simulink model "BatteryFarmTemplate"  (R2022b)
settings: Solver=VariableStepAuto  StartTime=0.0  StopTime=10.0  RelTol=1e-3  AbsTol=1e-3  EnableMultiTasking=on
libraries: ee_lib x242, sdl_lib x84, fl_lib x43
(part 1 of 5)
settings Model: Creator=Kimberly1!  LastModifiedBy=minar
settings SolverCC: AutoScaleAbsTol=off  AlgebraicLoopSolver=TrustRegion  MaxZcPerStep=1
settings DataIOCC: LimitDataPoints=on  MaxDataPoints=10000
settings OptimizationCC: LifeSpan=inf
settings DebuggingCC: UnconnectedInputMsg=warning  UnconnectedOutputMsg=warning  UnconnectedLineMsg=warning  AllowSymbolicDim=off  SFUnexpectedBacktrackingDiag=warning  SFNoUnconditionalDefaultTransitionDiag=warning  SFExecutionAtInitializationDiag=none  SFMachineParentedDataDiag=warning  ArithmeticOperatorsInVariantConditions=warning
settings ModelReferenceCC: EnableRefExpFcnMdlSchedulingChecks=on
settings SFSimCC: SimUseLocalCustomCode=off  CustomCodeUndefinedFunction=UseInterfaceOnly
settings RTWCC: RTWUseLocalCustomCode=off  DLArmComputeVersion=19.05
settings CodeAppCC: StateflowObjectComments=on
settings GRTTargetCC: TargetLangStandard=C89/C90 (ANSI)
settings ConfigComp: CovMetricSettings=dw  CovSaveCumulativeToWorkspaceVar=on  CovSaveSingleToWorkspaceVar=on  CovExternalEMLEnable=off  CovSFcnEnable=off
settings SimscapeCC: SimscapeLogType=all  SimscapeLogSimulationStatistics=on  SimscapeLogDataHistory=10000

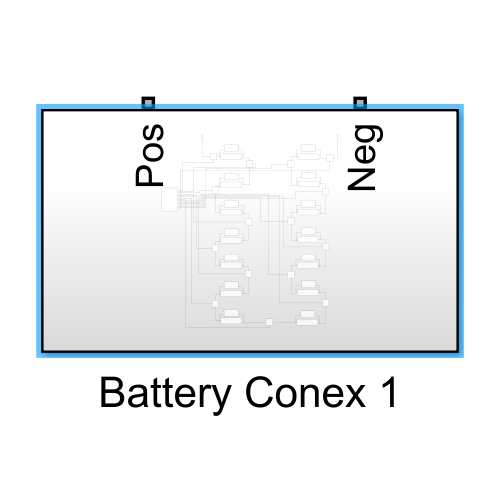
[thumbnail: Simulink's stored preview of the top-level diagram]
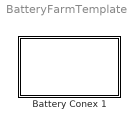
== system BatteryFarmTemplate ==
  Battery Conex 1 : Subsystem
      settings: PortSchema="{\"entries\":[{\"content\":{\"sides\":[{\"content\":{\"connectorIds\":[]},\"type\":\"ConnectorPlacement.EquallySpacedRectSide\",\"uuid\":\"048fa1c2-ad06-4d9f-ba7c-aee5a0b8c9f2\"},{\"content\":{\"connectorIds\":[],\"side\":\"RIGHT\"},\"type\":\"ConnectorPlacement.EquallySpacedRectSide\",\"uuid\":\"f15e2629-eceb-4a27-921b-d8c57562cf10\"},{\"content\":{\"connectorIds\":[\"LConn1\",\"LConn2\"],\"side\":\"TOP\"},\"type\":\"ConnectorPlacement.EquallySpacedRectSide\",\"uuid\":\"4da660f4-bcfa-4f4c-af01-21485ad5be59\"}]},\"type\":\"ConnectorPlacement.EquallySpacedConnector\",\"uuid\":\"40cf05ef-0db3-4ef6-b98b-cb586730e4e3\"}],\"packageUris\":[\"http://schema.mathworks.com/mf0/Connector/R2020b\"],\"version\":\"1.0\"}"

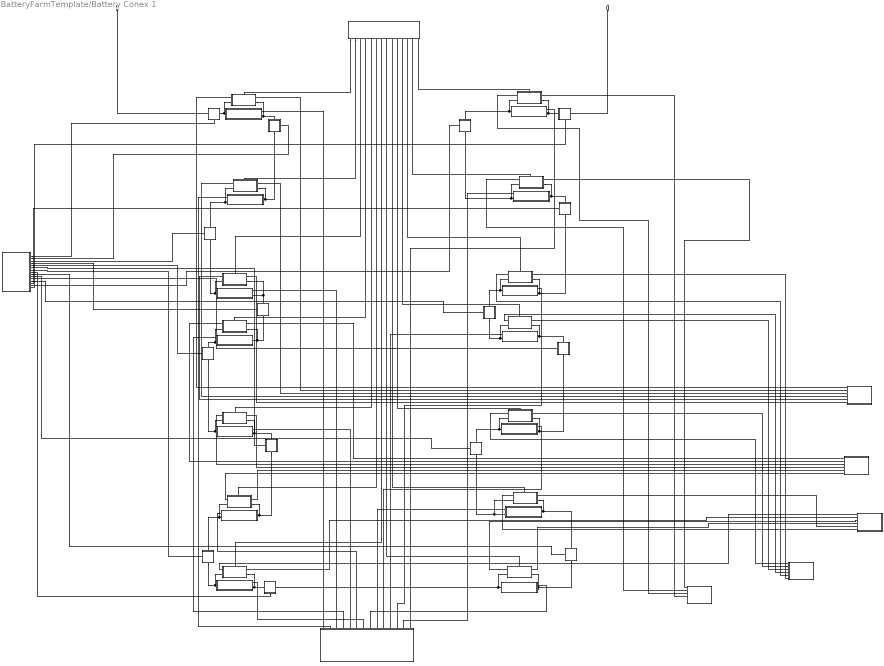
== system BatteryFarmTemplate/Battery Conex 1 ==
  Battery Charger 1 : Subsystem
  Battery Charger 2 : Subsystem
  Battery Charger 3 : Subsystem
  Battery Charger 4 : Subsystem
  Battery Charger 5 : Subsystem
  Battery Module 1 : Subsystem
  Battery Module 10 : Subsystem
  Battery Module 11 : Subsystem
  Battery Module 12 : Subsystem
  Battery Module 13 : Subsystem
  Battery Module 14 : Subsystem
  Battery Module 2 : Subsystem
  Battery Module 3 : Subsystem
  Battery Module 4 : Subsystem
  Battery Module 5 : Subsystem
  Battery Module 6 : Subsystem
  Battery Module 7 : Subsystem
  Battery Module 8 : Subsystem
  Battery Module 9 : Subsystem
  Busbar  SW 1 : Subsystem
      settings: PortSchema="{\"entries\":[{\"content\":{\"sides\":[{\"content\":{\"connectorIds\":[\"LConn1\"]},\"type\":\"ConnectorPlacement.EquallySpacedRectSide\",\"uuid\":\"9cfb2e44-9dde-4df9-b010-27803d6f9c91\"},{\"content\":{\"connectorIds\":[\"RConn1\"],\"side\":\"RIGHT\"},\"type\":\"ConnectorPlacement.EquallySpacedRectSide\",\"uuid\":\"4d379f47-42d8-42e3-9ed0-68a717690785\"},{\"content\":{\"connectorIds\":[],\"side\":\"TOP\"},\"type\":\"ConnectorPlacement.EquallySpacedRectSide\",\"uuid\":\"04b3dae9-36fd-4179-bf2b-fdf6296dfe4e\"},{\"content\":{\"connectorIds\":[\"RConn2\"],\"side\":\"BOTTOM\"},\"type\":\"ConnectorPlacement.EquallySpacedRectSide\",\"uuid\":\"a7774700-76cb-4b6b-87b6-7d3fc687af73\"}]},\"type\":\"ConnectorPlacement.EquallySpacedConnector\",\"uuid\":\"06353b4d-18ff-4963-8ee5-abf5474e4c27\"}],\"packageUris\":[\"http://schema.mathworks.com/mf0/Connector/R2020b\"],\"version\":\"1.0\"}"
  Busbar  SW 10 : Subsystem
      settings: PortSchema="{\"entries\":[{\"content\":{\"sides\":[{\"content\":{\"connectorIds\":[\"LConn1\"]},\"type\":\"ConnectorPlacement.EquallySpacedRectSide\",\"uuid\":\"9cfb2e44-9dde-4df9-b010-27803d6f9c91\"},{\"content\":{\"connectorIds\":[\"RConn1\"],\"side\":\"RIGHT\"},\"type\":\"ConnectorPlacement.EquallySpacedRectSide\",\"uuid\":\"4d379f47-42d8-42e3-9ed0-68a717690785\"},{\"content\":{\"connectorIds\":[],\"side\":\"TOP\"},\"type\":\"ConnectorPlacement.EquallySpacedRectSide\",\"uuid\":\"04b3dae9-36fd-4179-bf2b-fdf6296dfe4e\"},{\"content\":{\"connectorIds\":[\"RConn2\"],\"side\":\"BOTTOM\"},\"type\":\"ConnectorPlacement.EquallySpacedRectSide\",\"uuid\":\"a7774700-76cb-4b6b-87b6-7d3fc687af73\"}]},\"type\":\"ConnectorPlacement.EquallySpacedConnector\",\"uuid\":\"06353b4d-18ff-4963-8ee5-abf5474e4c27\"}],\"packageUris\":[\"http://schema.mathworks.com/mf0/Connector/R2020b\"],\"version\":\"1.0\"}"
  Busbar  SW 11 : Subsystem
      settings: PortSchema="{\"entries\":[{\"content\":{\"sides\":[{\"content\":{\"connectorIds\":[\"LConn1\"]},\"type\":\"ConnectorPlacement.EquallySpacedRectSide\",\"uuid\":\"9cfb2e44-9dde-4df9-b010-27803d6f9c91\"},{\"content\":{\"connectorIds\":[\"RConn1\"],\"side\":\"RIGHT\"},\"type\":\"ConnectorPlacement.EquallySpacedRectSide\",\"uuid\":\"4d379f47-42d8-42e3-9ed0-68a717690785\"},{\"content\":{\"connectorIds\":[],\"side\":\"TOP\"},\"type\":\"ConnectorPlacement.EquallySpacedRectSide\",\"uuid\":\"04b3dae9-36fd-4179-bf2b-fdf6296dfe4e\"},{\"content\":{\"connectorIds\":[\"RConn2\"],\"side\":\"BOTTOM\"},\"type\":\"ConnectorPlacement.EquallySpacedRectSide\",\"uuid\":\"a7774700-76cb-4b6b-87b6-7d3fc687af73\"}]},\"type\":\"ConnectorPlacement.EquallySpacedConnector\",\"uuid\":\"06353b4d-18ff-4963-8ee5-abf5474e4c27\"}],\"packageUris\":[\"http://schema.mathworks.com/mf0/Connector/R2020b\"],\"version\":\"1.0\"}"
  Busbar  SW 12 : Subsystem
      settings: PortSchema="{\"entries\":[{\"content\":{\"sides\":[{\"content\":{\"connectorIds\":[\"LConn1\"]},\"type\":\"ConnectorPlacement.EquallySpacedRectSide\",\"uuid\":\"9cfb2e44-9dde-4df9-b010-27803d6f9c91\"},{\"content\":{\"connectorIds\":[\"RConn1\"],\"side\":\"RIGHT\"},\"type\":\"ConnectorPlacement.EquallySpacedRectSide\",\"uuid\":\"4d379f47-42d8-42e3-9ed0-68a717690785\"},{\"content\":{\"connectorIds\":[],\"side\":\"TOP\"},\"type\":\"ConnectorPlacement.EquallySpacedRectSide\",\"uuid\":\"04b3dae9-36fd-4179-bf2b-fdf6296dfe4e\"},{\"content\":{\"connectorIds\":[\"RConn2\"],\"side\":\"BOTTOM\"},\"type\":\"ConnectorPlacement.EquallySpacedRectSide\",\"uuid\":\"a7774700-76cb-4b6b-87b6-7d3fc687af73\"}]},\"type\":\"ConnectorPlacement.EquallySpacedConnector\",\"uuid\":\"06353b4d-18ff-4963-8ee5-abf5474e4c27\"}],\"packageUris\":[\"http://schema.mathworks.com/mf0/Connector/R2020b\"],\"version\":\"1.0\"}"
  Busbar  SW 13 : Subsystem
      settings: PortSchema="{\"entries\":[{\"content\":{\"sides\":[{\"content\":{\"connectorIds\":[\"LConn1\"]},\"type\":\"ConnectorPlacement.EquallySpacedRectSide\",\"uuid\":\"9cfb2e44-9dde-4df9-b010-27803d6f9c91\"},{\"content\":{\"connectorIds\":[\"RConn1\"],\"side\":\"RIGHT\"},\"type\":\"ConnectorPlacement.EquallySpacedRectSide\",\"uuid\":\"4d379f47-42d8-42e3-9ed0-68a717690785\"},{\"content\":{\"connectorIds\":[],\"side\":\"TOP\"},\"type\":\"ConnectorPlacement.EquallySpacedRectSide\",\"uuid\":\"04b3dae9-36fd-4179-bf2b-fdf6296dfe4e\"},{\"content\":{\"connectorIds\":[\"RConn2\"],\"side\":\"BOTTOM\"},\"type\":\"ConnectorPlacement.EquallySpacedRectSide\",\"uuid\":\"a7774700-76cb-4b6b-87b6-7d3fc687af73\"}]},\"type\":\"ConnectorPlacement.EquallySpacedConnector\",\"uuid\":\"06353b4d-18ff-4963-8ee5-abf5474e4c27\"}],\"packageUris\":[\"http://schema.mathworks.com/mf0/Connector/R2020b\"],\"version\":\"1.0\"}"
  Busbar  SW 14 : Subsystem
      settings: PortSchema="{\"entries\":[{\"content\":{\"sides\":[{\"content\":{\"connectorIds\":[\"LConn1\"]},\"type\":\"ConnectorPlacement.EquallySpacedRectSide\",\"uuid\":\"9cfb2e44-9dde-4df9-b010-27803d6f9c91\"},{\"content\":{\"connectorIds\":[\"RConn1\"],\"side\":\"RIGHT\"},\"type\":\"ConnectorPlacement.EquallySpacedRectSide\",\"uuid\":\"4d379f47-42d8-42e3-9ed0-68a717690785\"},{\"content\":{\"connectorIds\":[],\"side\":\"TOP\"},\"type\":\"ConnectorPlacement.EquallySpacedRectSide\",\"uuid\":\"04b3dae9-36fd-4179-bf2b-fdf6296dfe4e\"},{\"content\":{\"connectorIds\":[\"RConn2\"],\"side\":\"BOTTOM\"},\"type\":\"ConnectorPlacement.EquallySpacedRectSide\",\"uuid\":\"a7774700-76cb-4b6b-87b6-7d3fc687af73\"}]},\"type\":\"ConnectorPlacement.EquallySpacedConnector\",\"uuid\":\"06353b4d-18ff-4963-8ee5-abf5474e4c27\"}],\"packageUris\":[\"http://schema.mathworks.com/mf0/Connector/R2020b\"],\"version\":\"1.0\"}"
  Busbar  SW 15 : Subsystem
      settings: PortSchema="{\"entries\":[{\"content\":{\"sides\":[{\"content\":{\"connectorIds\":[\"LConn1\"]},\"type\":\"ConnectorPlacement.EquallySpacedRectSide\",\"uuid\":\"9cfb2e44-9dde-4df9-b010-27803d6f9c91\"},{\"content\":{\"connectorIds\":[\"RConn1\"],\"side\":\"RIGHT\"},\"type\":\"ConnectorPlacement.EquallySpacedRectSide\",\"uuid\":\"4d379f47-42d8-42e3-9ed0-68a717690785\"},{\"content\":{\"connectorIds\":[],\"side\":\"TOP\"},\"type\":\"ConnectorPlacement.EquallySpacedRectSide\",\"uuid\":\"04b3dae9-36fd-4179-bf2b-fdf6296dfe4e\"},{\"content\":{\"connectorIds\":[\"RConn2\"],\"side\":\"BOTTOM\"},\"type\":\"ConnectorPlacement.EquallySpacedRectSide\",\"uuid\":\"a7774700-76cb-4b6b-87b6-7d3fc687af73\"}]},\"type\":\"ConnectorPlacement.EquallySpacedConnector\",\"uuid\":\"06353b4d-18ff-4963-8ee5-abf5474e4c27\"}],\"packageUris\":[\"http://schema.mathworks.com/mf0/Connector/R2020b\"],\"version\":\"1.0\"}"
  Busbar  SW 2 : Subsystem
      settings: PortSchema="{\"entries\":[{\"content\":{\"sides\":[{\"content\":{\"connectorIds\":[\"LConn1\"]},\"type\":\"ConnectorPlacement.EquallySpacedRectSide\",\"uuid\":\"9cfb2e44-9dde-4df9-b010-27803d6f9c91\"},{\"content\":{\"connectorIds\":[\"RConn1\"],\"side\":\"RIGHT\"},\"type\":\"ConnectorPlacement.EquallySpacedRectSide\",\"uuid\":\"4d379f47-42d8-42e3-9ed0-68a717690785\"},{\"content\":{\"connectorIds\":[],\"side\":\"TOP\"},\"type\":\"ConnectorPlacement.EquallySpacedRectSide\",\"uuid\":\"04b3dae9-36fd-4179-bf2b-fdf6296dfe4e\"},{\"content\":{\"connectorIds\":[\"RConn2\"],\"side\":\"BOTTOM\"},\"type\":\"ConnectorPlacement.EquallySpacedRectSide\",\"uuid\":\"a7774700-76cb-4b6b-87b6-7d3fc687af73\"}]},\"type\":\"ConnectorPlacement.EquallySpacedConnector\",\"uuid\":\"06353b4d-18ff-4963-8ee5-abf5474e4c27\"}],\"packageUris\":[\"http://schema.mathworks.com/mf0/Connector/R2020b\"],\"version\":\"1.0\"}"
  Busbar  SW 3 : Subsystem
      settings: PortSchema="{\"entries\":[{\"content\":{\"sides\":[{\"content\":{\"connectorIds\":[\"LConn1\"]},\"type\":\"ConnectorPlacement.EquallySpacedRectSide\",\"uuid\":\"9cfb2e44-9dde-4df9-b010-27803d6f9c91\"},{\"content\":{\"connectorIds\":[\"RConn1\"],\"side\":\"RIGHT\"},\"type\":\"ConnectorPlacement.EquallySpacedRectSide\",\"uuid\":\"4d379f47-42d8-42e3-9ed0-68a717690785\"},{\"content\":{\"connectorIds\":[],\"side\":\"TOP\"},\"type\":\"ConnectorPlacement.EquallySpacedRectSide\",\"uuid\":\"04b3dae9-36fd-4179-bf2b-fdf6296dfe4e\"},{\"content\":{\"connectorIds\":[\"RConn2\"],\"side\":\"BOTTOM\"},\"type\":\"ConnectorPlacement.EquallySpacedRectSide\",\"uuid\":\"a7774700-76cb-4b6b-87b6-7d3fc687af73\"}]},\"type\":\"ConnectorPlacement.EquallySpacedConnector\",\"uuid\":\"06353b4d-18ff-4963-8ee5-abf5474e4c27\"}],\"packageUris\":[\"http://schema.mathworks.com/mf0/Connector/R2020b\"],\"version\":\"1.0\"}"
  Busbar  SW 4 : Subsystem
      settings: PortSchema="{\"entries\":[{\"content\":{\"sides\":[{\"content\":{\"connectorIds\":[\"LConn1\"]},\"type\":\"ConnectorPlacement.EquallySpacedRectSide\",\"uuid\":\"9cfb2e44-9dde-4df9-b010-27803d6f9c91\"},{\"content\":{\"connectorIds\":[\"RConn1\"],\"side\":\"RIGHT\"},\"type\":\"ConnectorPlacement.EquallySpacedRectSide\",\"uuid\":\"4d379f47-42d8-42e3-9ed0-68a717690785\"},{\"content\":{\"connectorIds\":[],\"side\":\"TOP\"},\"type\":\"ConnectorPlacement.EquallySpacedRectSide\",\"uuid\":\"04b3dae9-36fd-4179-bf2b-fdf6296dfe4e\"},{\"content\":{\"connectorIds\":[\"RConn2\"],\"side\":\"BOTTOM\"},\"type\":\"ConnectorPlacement.EquallySpacedRectSide\",\"uuid\":\"a7774700-76cb-4b6b-87b6-7d3fc687af73\"}]},\"type\":\"ConnectorPlacement.EquallySpacedConnector\",\"uuid\":\"06353b4d-18ff-4963-8ee5-abf5474e4c27\"}],\"packageUris\":[\"http://schema.mathworks.com/mf0/Connector/R2020b\"],\"version\":\"1.0\"}"
  Busbar  SW 5 : Subsystem
      settings: PortSchema="{\"entries\":[{\"content\":{\"sides\":[{\"content\":{\"connectorIds\":[\"LConn1\"]},\"type\":\"ConnectorPlacement.EquallySpacedRectSide\",\"uuid\":\"9cfb2e44-9dde-4df9-b010-27803d6f9c91\"},{\"content\":{\"connectorIds\":[\"RConn1\"],\"side\":\"RIGHT\"},\"type\":\"ConnectorPlacement.EquallySpacedRectSide\",\"uuid\":\"4d379f47-42d8-42e3-9ed0-68a717690785\"},{\"content\":{\"connectorIds\":[],\"side\":\"TOP\"},\"type\":\"ConnectorPlacement.EquallySpacedRectSide\",\"uuid\":\"04b3dae9-36fd-4179-bf2b-fdf6296dfe4e\"},{\"content\":{\"connectorIds\":[\"RConn2\"],\"side\":\"BOTTOM\"},\"type\":\"ConnectorPlacement.EquallySpacedRectSide\",\"uuid\":\"a7774700-76cb-4b6b-87b6-7d3fc687af73\"}]},\"type\":\"ConnectorPlacement.EquallySpacedConnector\",\"uuid\":\"06353b4d-18ff-4963-8ee5-abf5474e4c27\"}],\"packageUris\":[\"http://schema.mathworks.com/mf0/Connector/R2020b\"],\"version\":\"1.0\"}"
  Busbar  SW 6 : Subsystem
      settings: PortSchema="{\"entries\":[{\"content\":{\"sides\":[{\"content\":{\"connectorIds\":[\"LConn1\"]},\"type\":\"ConnectorPlacement.EquallySpacedRectSide\",\"uuid\":\"9cfb2e44-9dde-4df9-b010-27803d6f9c91\"},{\"content\":{\"connectorIds\":[\"RConn1\"],\"side\":\"RIGHT\"},\"type\":\"ConnectorPlacement.EquallySpacedRectSide\",\"uuid\":\"4d379f47-42d8-42e3-9ed0-68a717690785\"},{\"content\":{\"connectorIds\":[],\"side\":\"TOP\"},\"type\":\"ConnectorPlacement.EquallySpacedRectSide\",\"uuid\":\"04b3dae9-36fd-4179-bf2b-fdf6296dfe4e\"},{\"content\":{\"connectorIds\":[\"RConn2\"],\"side\":\"BOTTOM\"},\"type\":\"ConnectorPlacement.EquallySpacedRectSide\",\"uuid\":\"a7774700-76cb-4b6b-87b6-7d3fc687af73\"}]},\"type\":\"ConnectorPlacement.EquallySpacedConnector\",\"uuid\":\"06353b4d-18ff-4963-8ee5-abf5474e4c27\"}],\"packageUris\":[\"http://schema.mathworks.com/mf0/Connector/R2020b\"],\"version\":\"1.0\"}"
  Busbar  SW 7 : Subsystem
      settings: PortSchema="{\"entries\":[{\"content\":{\"sides\":[{\"content\":{\"connectorIds\":[\"LConn1\"]},\"type\":\"ConnectorPlacement.EquallySpacedRectSide\",\"uuid\":\"9cfb2e44-9dde-4df9-b010-27803d6f9c91\"},{\"content\":{\"connectorIds\":[\"RConn1\"],\"side\":\"RIGHT\"},\"type\":\"ConnectorPlacement.EquallySpacedRectSide\",\"uuid\":\"4d379f47-42d8-42e3-9ed0-68a717690785\"},{\"content\":{\"connectorIds\":[],\"side\":\"TOP\"},\"type\":\"ConnectorPlacement.EquallySpacedRectSide\",\"uuid\":\"04b3dae9-36fd-4179-bf2b-fdf6296dfe4e\"},{\"content\":{\"connectorIds\":[\"RConn2\"],\"side\":\"BOTTOM\"},\"type\":\"ConnectorPlacement.EquallySpacedRectSide\",\"uuid\":\"a7774700-76cb-4b6b-87b6-7d3fc687af73\"}]},\"type\":\"ConnectorPlacement.EquallySpacedConnector\",\"uuid\":\"06353b4d-18ff-4963-8ee5-abf5474e4c27\"}],\"packageUris\":[\"http://schema.mathworks.com/mf0/Connector/R2020b\"],\"version\":\"1.0\"}"
  Busbar  SW 8 : Subsystem
      settings: PortSchema="{\"entries\":[{\"content\":{\"sides\":[{\"content\":{\"connectorIds\":[\"LConn1\"]},\"type\":\"ConnectorPlacement.EquallySpacedRectSide\",\"uuid\":\"9cfb2e44-9dde-4df9-b010-27803d6f9c91\"},{\"content\":{\"connectorIds\":[\"RConn1\"],\"side\":\"RIGHT\"},\"type\":\"ConnectorPlacement.EquallySpacedRectSide\",\"uuid\":\"4d379f47-42d8-42e3-9ed0-68a717690785\"},{\"content\":{\"connectorIds\":[],\"side\":\"TOP\"},\"type\":\"ConnectorPlacement.EquallySpacedRectSide\",\"uuid\":\"04b3dae9-36fd-4179-bf2b-fdf6296dfe4e\"},{\"content\":{\"connectorIds\":[\"RConn2\"],\"side\":\"BOTTOM\"},\"type\":\"ConnectorPlacement.EquallySpacedRectSide\",\"uuid\":\"a7774700-76cb-4b6b-87b6-7d3fc687af73\"}]},\"type\":\"ConnectorPlacement.EquallySpacedConnector\",\"uuid\":\"06353b4d-18ff-4963-8ee5-abf5474e4c27\"}],\"packageUris\":[\"http://schema.mathworks.com/mf0/Connector/R2020b\"],\"version\":\"1.0\"}"
  Busbar  SW 9 : Subsystem
      settings: PortSchema="{\"entries\":[{\"content\":{\"sides\":[{\"content\":{\"connectorIds\":[\"LConn1\"]},\"type\":\"ConnectorPlacement.EquallySpacedRectSide\",\"uuid\":\"9cfb2e44-9dde-4df9-b010-27803d6f9c91\"},{\"content\":{\"connectorIds\":[\"RConn1\"],\"side\":\"RIGHT\"},\"type\":\"ConnectorPlacement.EquallySpacedRectSide\",\"uuid\":\"4d379f47-42d8-42e3-9ed0-68a717690785\"},{\"content\":{\"connectorIds\":[],\"side\":\"TOP\"},\"type\":\"ConnectorPlacement.EquallySpacedRectSide\",\"uuid\":\"04b3dae9-36fd-4179-bf2b-fdf6296dfe4e\"},{\"content\":{\"connectorIds\":[\"RConn2\"],\"side\":\"BOTTOM\"},\"type\":\"ConnectorPlacement.EquallySpacedRectSide\",\"uuid\":\"a7774700-76cb-4b6b-87b6-7d3fc687af73\"}]},\"type\":\"ConnectorPlacement.EquallySpacedConnector\",\"uuid\":\"06353b4d-18ff-4963-8ee5-abf5474e4c27\"}],\"packageUris\":[\"http://schema.mathworks.com/mf0/Connector/R2020b\"],\"version\":\"1.0\"}"
  Discharge Relay Controller : Subsystem
  Parallel Charge 1 : Subsystem
      settings: PortSchema="{\"entries\":[{\"content\":{\"sides\":[{\"content\":{\"connectorIds\":[\"LConn1\",\"LConn2\"]},\"type\":\"ConnectorPlacement.EquallySpacedRectSide\",\"uuid\":\"92b66880-3ab5-48ec-aaf6-0b390f6e8e6c\"},{\"content\":{\"connectorIds\":[\"RConn1\",\"RConn2\"],\"side\":\"RIGHT\"},\"type\":\"ConnectorPlacement.EquallySpacedRectSide\",\"uuid\":\"e85905ce-1804-41fb-a21c-30ce2b9855cf\"},{\"content\":{\"connectorIds\":[\"LConn3\"],\"side\":\"TOP\"},\"type\":\"ConnectorPlacement.EquallySpacedRectSide\",\"uuid\":\"eff338fa-75bd-4848-9daa-8afb385e699a\"}]},\"type\":\"ConnectorPlacement.EquallySpacedConnector\",\"uuid\":\"4f6beb8f-1b0c-4e7d-9e2e-53f134c38bf2\"}],\"packageUris\":[\"http://schema.mathworks.com/mf0/Connector/R2020b\"],\"version\":\"1.0\"}"
  Parallel Charge 10 : Subsystem
      settings: PortSchema="{\"entries\":[{\"content\":{\"sides\":[{\"content\":{\"connectorIds\":[\"LConn1\",\"LConn2\"]},\"type\":\"ConnectorPlacement.EquallySpacedRectSide\",\"uuid\":\"92b66880-3ab5-48ec-aaf6-0b390f6e8e6c\"},{\"content\":{\"connectorIds\":[\"RConn1\",\"RConn2\"],\"side\":\"RIGHT\"},\"type\":\"ConnectorPlacement.EquallySpacedRectSide\",\"uuid\":\"e85905ce-1804-41fb-a21c-30ce2b9855cf\"},{\"content\":{\"connectorIds\":[\"LConn3\"],\"side\":\"TOP\"},\"type\":\"ConnectorPlacement.EquallySpacedRectSide\",\"uuid\":\"eff338fa-75bd-4848-9daa-8afb385e699a\"}]},\"type\":\"ConnectorPlacement.EquallySpacedConnector\",\"uuid\":\"4f6beb8f-1b0c-4e7d-9e2e-53f134c38bf2\"}],\"packageUris\":[\"http://schema.mathworks.com/mf0/Connector/R2020b\"],\"version\":\"1.0\"}"
  Parallel Charge 11 : Subsystem
      settings: PortSchema="{\"entries\":[{\"content\":{\"sides\":[{\"content\":{\"connectorIds\":[\"LConn1\",\"LConn2\"]},\"type\":\"ConnectorPlacement.EquallySpacedRectSide\",\"uuid\":\"92b66880-3ab5-48ec-aaf6-0b390f6e8e6c\"},{\"content\":{\"connectorIds\":[\"RConn1\",\"RConn2\"],\"side\":\"RIGHT\"},\"type\":\"ConnectorPlacement.EquallySpacedRectSide\",\"uuid\":\"e85905ce-1804-41fb-a21c-30ce2b9855cf\"},{\"content\":{\"connectorIds\":[\"LConn3\"],\"side\":\"TOP\"},\"type\":\"ConnectorPlacement.EquallySpacedRectSide\",\"uuid\":\"eff338fa-75bd-4848-9daa-8afb385e699a\"}]},\"type\":\"ConnectorPlacement.EquallySpacedConnector\",\"uuid\":\"4f6beb8f-1b0c-4e7d-9e2e-53f134c38bf2\"}],\"packageUris\":[\"http://schema.mathworks.com/mf0/Connector/R2020b\"],\"version\":\"1.0\"}"
  Parallel Charge 12 : Subsystem
      settings: PortSchema="{\"entries\":[{\"content\":{\"sides\":[{\"content\":{\"connectorIds\":[\"LConn1\",\"LConn2\"]},\"type\":\"ConnectorPlacement.EquallySpacedRectSide\",\"uuid\":\"92b66880-3ab5-48ec-aaf6-0b390f6e8e6c\"},{\"content\":{\"connectorIds\":[\"RConn1\",\"RConn2\"],\"side\":\"RIGHT\"},\"type\":\"ConnectorPlacement.EquallySpacedRectSide\",\"uuid\":\"e85905ce-1804-41fb-a21c-30ce2b9855cf\"},{\"content\":{\"connectorIds\":[\"LConn3\"],\"side\":\"TOP\"},\"type\":\"ConnectorPlacement.EquallySpacedRectSide\",\"uuid\":\"eff338fa-75bd-4848-9daa-8afb385e699a\"}]},\"type\":\"ConnectorPlacement.EquallySpacedConnector\",\"uuid\":\"4f6beb8f-1b0c-4e7d-9e2e-53f134c38bf2\"}],\"packageUris\":[\"http://schema.mathworks.com/mf0/Connector/R2020b\"],\"version\":\"1.0\"}"
  Parallel Charge 13 : Subsystem
      settings: PortSchema="{\"entries\":[{\"content\":{\"sides\":[{\"content\":{\"connectorIds\":[\"LConn1\",\"LConn2\"]},\"type\":\"ConnectorPlacement.EquallySpacedRectSide\",\"uuid\":\"92b66880-3ab5-48ec-aaf6-0b390f6e8e6c\"},{\"content\":{\"connectorIds\":[\"RConn1\",\"RConn2\"],\"side\":\"RIGHT\"},\"type\":\"ConnectorPlacement.EquallySpacedRectSide\",\"uuid\":\"e85905ce-1804-41fb-a21c-30ce2b9855cf\"},{\"content\":{\"connectorIds\":[\"LConn3\"],\"side\":\"TOP\"},\"type\":\"ConnectorPlacement.EquallySpacedRectSide\",\"uuid\":\"eff338fa-75bd-4848-9daa-8afb385e699a\"}]},\"type\":\"ConnectorPlacement.EquallySpacedConnector\",\"uuid\":\"4f6beb8f-1b0c-4e7d-9e2e-53f134c38bf2\"}],\"packageUris\":[\"http://schema.mathworks.com/mf0/Connector/R2020b\"],\"version\":\"1.0\"}"
  Parallel Charge 14 : Subsystem
      settings: PortSchema="{\"entries\":[{\"content\":{\"sides\":[{\"content\":{\"connectorIds\":[\"LConn1\",\"LConn2\"]},\"type\":\"ConnectorPlacement.EquallySpacedRectSide\",\"uuid\":\"92b66880-3ab5-48ec-aaf6-0b390f6e8e6c\"},{\"content\":{\"connectorIds\":[\"RConn1\",\"RConn2\"],\"side\":\"RIGHT\"},\"type\":\"ConnectorPlacement.EquallySpacedRectSide\",\"uuid\":\"e85905ce-1804-41fb-a21c-30ce2b9855cf\"},{\"content\":{\"connectorIds\":[\"LConn3\"],\"side\":\"TOP\"},\"type\":\"ConnectorPlacement.EquallySpacedRectSide\",\"uuid\":\"eff338fa-75bd-4848-9daa-8afb385e699a\"}]},\"type\":\"ConnectorPlacement.EquallySpacedConnector\",\"uuid\":\"4f6beb8f-1b0c-4e7d-9e2e-53f134c38bf2\"}],\"packageUris\":[\"http://schema.mathworks.com/mf0/Connector/R2020b\"],\"version\":\"1.0\"}"
  Parallel Charge 2 : Subsystem
      settings: PortSchema="{\"entries\":[{\"content\":{\"sides\":[{\"content\":{\"connectorIds\":[\"LConn1\",\"LConn2\"]},\"type\":\"ConnectorPlacement.EquallySpacedRectSide\",\"uuid\":\"92b66880-3ab5-48ec-aaf6-0b390f6e8e6c\"},{\"content\":{\"connectorIds\":[\"RConn1\",\"RConn2\"],\"side\":\"RIGHT\"},\"type\":\"ConnectorPlacement.EquallySpacedRectSide\",\"uuid\":\"e85905ce-1804-41fb-a21c-30ce2b9855cf\"},{\"content\":{\"connectorIds\":[\"LConn3\"],\"side\":\"TOP\"},\"type\":\"ConnectorPlacement.EquallySpacedRectSide\",\"uuid\":\"eff338fa-75bd-4848-9daa-8afb385e699a\"}]},\"type\":\"ConnectorPlacement.EquallySpacedConnector\",\"uuid\":\"4f6beb8f-1b0c-4e7d-9e2e-53f134c38bf2\"}],\"packageUris\":[\"http://schema.mathworks.com/mf0/Connector/R2020b\"],\"version\":\"1.0\"}"
  Parallel Charge 3 : Subsystem
      settings: PortSchema="{\"entries\":[{\"content\":{\"sides\":[{\"content\":{\"connectorIds\":[\"LConn1\",\"LConn2\"]},\"type\":\"ConnectorPlacement.EquallySpacedRectSide\",\"uuid\":\"92b66880-3ab5-48ec-aaf6-0b390f6e8e6c\"},{\"content\":{\"connectorIds\":[\"RConn1\",\"RConn2\"],\"side\":\"RIGHT\"},\"type\":\"ConnectorPlacement.EquallySpacedRectSide\",\"uuid\":\"e85905ce-1804-41fb-a21c-30ce2b9855cf\"},{\"content\":{\"connectorIds\":[\"LConn3\"],\"side\":\"TOP\"},\"type\":\"ConnectorPlacement.EquallySpacedRectSide\",\"uuid\":\"eff338fa-75bd-4848-9daa-8afb385e699a\"}]},\"type\":\"ConnectorPlacement.EquallySpacedConnector\",\"uuid\":\"4f6beb8f-1b0c-4e7d-9e2e-53f134c38bf2\"}],\"packageUris\":[\"http://schema.mathworks.com/mf0/Connector/R2020b\"],\"version\":\"1.0\"}"
  Parallel Charge 4 : Subsystem
      settings: PortSchema="{\"entries\":[{\"content\":{\"sides\":[{\"content\":{\"connectorIds\":[\"LConn1\",\"LConn2\"]},\"type\":\"ConnectorPlacement.EquallySpacedRectSide\",\"uuid\":\"92b66880-3ab5-48ec-aaf6-0b390f6e8e6c\"},{\"content\":{\"connectorIds\":[\"RConn1\",\"RConn2\"],\"side\":\"RIGHT\"},\"type\":\"ConnectorPlacement.EquallySpacedRectSide\",\"uuid\":\"e85905ce-1804-41fb-a21c-30ce2b9855cf\"},{\"content\":{\"connectorIds\":[\"LConn3\"],\"side\":\"TOP\"},\"type\":\"ConnectorPlacement.EquallySpacedRectSide\",\"uuid\":\"eff338fa-75bd-4848-9daa-8afb385e699a\"}]},\"type\":\"ConnectorPlacement.EquallySpacedConnector\",\"uuid\":\"4f6beb8f-1b0c-4e7d-9e2e-53f134c38bf2\"}],\"packageUris\":[\"http://schema.mathworks.com/mf0/Connector/R2020b\"],\"version\":\"1.0\"}"
  Parallel Charge 5 : Subsystem
      settings: PortSchema="{\"entries\":[{\"content\":{\"sides\":[{\"content\":{\"connectorIds\":[\"LConn1\",\"LConn2\"]},\"type\":\"ConnectorPlacement.EquallySpacedRectSide\",\"uuid\":\"92b66880-3ab5-48ec-aaf6-0b390f6e8e6c\"},{\"content\":{\"connectorIds\":[\"RConn1\",\"RConn2\"],\"side\":\"RIGHT\"},\"type\":\"ConnectorPlacement.EquallySpacedRectSide\",\"uuid\":\"e85905ce-1804-41fb-a21c-30ce2b9855cf\"},{\"content\":{\"connectorIds\":[\"LConn3\"],\"side\":\"TOP\"},\"type\":\"ConnectorPlacement.EquallySpacedRectSide\",\"uuid\":\"eff338fa-75bd-4848-9daa-8afb385e699a\"}]},\"type\":\"ConnectorPlacement.EquallySpacedConnector\",\"uuid\":\"4f6beb8f-1b0c-4e7d-9e2e-53f134c38bf2\"}],\"packageUris\":[\"http://schema.mathworks.com/mf0/Connector/R2020b\"],\"version\":\"1.0\"}"
  Parallel Charge 6 : Subsystem
      settings: PortSchema="{\"entries\":[{\"content\":{\"sides\":[{\"content\":{\"connectorIds\":[\"LConn1\",\"LConn2\"]},\"type\":\"ConnectorPlacement.EquallySpacedRectSide\",\"uuid\":\"92b66880-3ab5-48ec-aaf6-0b390f6e8e6c\"},{\"content\":{\"connectorIds\":[\"RConn1\",\"RConn2\"],\"side\":\"RIGHT\"},\"type\":\"ConnectorPlacement.EquallySpacedRectSide\",\"uuid\":\"e85905ce-1804-41fb-a21c-30ce2b9855cf\"},{\"content\":{\"connectorIds\":[\"LConn3\"],\"side\":\"TOP\"},\"type\":\"ConnectorPlacement.EquallySpacedRectSide\",\"uuid\":\"eff338fa-75bd-4848-9daa-8afb385e699a\"}]},\"type\":\"ConnectorPlacement.EquallySpacedConnector\",\"uuid\":\"4f6beb8f-1b0c-4e7d-9e2e-53f134c38bf2\"}],\"packageUris\":[\"http://schema.mathworks.com/mf0/Connector/R2020b\"],\"version\":\"1.0\"}"
  Parallel Charge 7 : Subsystem
      settings: PortSchema="{\"entries\":[{\"content\":{\"sides\":[{\"content\":{\"connectorIds\":[\"LConn1\",\"LConn2\"]},\"type\":\"ConnectorPlacement.EquallySpacedRectSide\",\"uuid\":\"92b66880-3ab5-48ec-aaf6-0b390f6e8e6c\"},{\"content\":{\"connectorIds\":[\"RConn1\",\"RConn2\"],\"side\":\"RIGHT\"},\"type\":\"ConnectorPlacement.EquallySpacedRectSide\",\"uuid\":\"e85905ce-1804-41fb-a21c-30ce2b9855cf\"},{\"content\":{\"connectorIds\":[\"LConn3\"],\"side\":\"TOP\"},\"type\":\"ConnectorPlacement.EquallySpacedRectSide\",\"uuid\":\"eff338fa-75bd-4848-9daa-8afb385e699a\"}]},\"type\":\"ConnectorPlacement.EquallySpacedConnector\",\"uuid\":\"4f6beb8f-1b0c-4e7d-9e2e-53f134c38bf2\"}],\"packageUris\":[\"http://schema.mathworks.com/mf0/Connector/R2020b\"],\"version\":\"1.0\"}"
  Parallel Charge 8 : Subsystem
      settings: PortSchema="{\"entries\":[{\"content\":{\"sides\":[{\"content\":{\"connectorIds\":[\"LConn1\",\"LConn2\"]},\"type\":\"ConnectorPlacement.EquallySpacedRectSide\",\"uuid\":\"92b66880-3ab5-48ec-aaf6-0b390f6e8e6c\"},{\"content\":{\"connectorIds\":[\"RConn1\",\"RConn2\"],\"side\":\"RIGHT\"},\"type\":\"ConnectorPlacement.EquallySpacedRectSide\",\"uuid\":\"e85905ce-1804-41fb-a21c-30ce2b9855cf\"},{\"content\":{\"connectorIds\":[\"LConn3\"],\"side\":\"TOP\"},\"type\":\"ConnectorPlacement.EquallySpacedRectSide\",\"uuid\":\"eff338fa-75bd-4848-9daa-8afb385e699a\"}]},\"type\":\"ConnectorPlacement.EquallySpacedConnector\",\"uuid\":\"4f6beb8f-1b0c-4e7d-9e2e-53f134c38bf2\"}],\"packageUris\":[\"http://schema.mathworks.com/mf0/Connector/R2020b\"],\"version\":\"1.0\"}"
  Parallel Charge 9 : Subsystem
      settings: PortSchema="{\"entries\":[{\"content\":{\"sides\":[{\"content\":{\"connectorIds\":[\"LConn1\",\"LConn2\"]},\"type\":\"ConnectorPlacement.EquallySpacedRectSide\",\"uuid\":\"92b66880-3ab5-48ec-aaf6-0b390f6e8e6c\"},{\"content\":{\"connectorIds\":[\"RConn1\",\"RConn2\"],\"side\":\"RIGHT\"},\"type\":\"ConnectorPlacement.EquallySpacedRectSide\",\"uuid\":\"e85905ce-1804-41fb-a21c-30ce2b9855cf\"},{\"content\":{\"connectorIds\":[\"LConn3\"],\"side\":\"TOP\"},\"type\":\"ConnectorPlacement.EquallySpacedRectSide\",\"uuid\":\"eff338fa-75bd-4848-9daa-8afb385e699a\"}]},\"type\":\"ConnectorPlacement.EquallySpacedConnector\",\"uuid\":\"4f6beb8f-1b0c-4e7d-9e2e-53f134c38bf2\"}],\"packageUris\":[\"http://schema.mathworks.com/mf0/Connector/R2020b\"],\"version\":\"1.0\"}"
  Parallel Relay Control : Subsystem
      settings: PortSchema="{\"entries\":[{\"content\":{\"sides\":[{\"content\":{\"connectorIds\":[]},\"type\":\"ConnectorPlacement.EquallySpacedRectSide\",\"uuid\":\"4757950b-f271-4edd-ae1d-136b19e50fcd\"},{\"content\":{\"connectorIds\":[],\"side\":\"RIGHT\"},\"type\":\"ConnectorPlacement.EquallySpacedRectSide\",\"uuid\":\"8cc8957e-d6c5-4df5-9611-0740750c5ab9\"},{\"content\":{\"connectorIds\":[],\"side\":\"TOP\"},\"type\":\"ConnectorPlacement.EquallySpacedRectSide\",\"uuid\":\"3bcc0884-f747-4e8b-a0cd-197e86d0460c\"},{\"content\":{\"connectorIds\":[\"RConn1\",\"RConn2\",\"RConn3\",\"RConn4\",\"RConn5\",\"RConn6\",\"RConn7\",\"RConn8\",\"RConn9\",\"RConn10\",\"RConn11\",\"RConn12\",\"RConn13\",\"RConn14\"],\"side\":\"BOTTOM\"},\"type\":\"ConnectorPlacement.EquallySpacedRectSide\",\"uuid\":\"a644c9ca-9e72-4d50-a6f0-17ec36fe7169\"}]},\"type\":\"ConnectorPlacement.EquallySpacedConnector\",\"uuid\":\"77d50f54-44ae-48af-989c-d8b33832f1b0\"}],\"packageUris\":[\"http://schema.mathworks.com/mf0/Connector/R2020b\"],\"version\":\"1.0\"}"
  Thermal Control : Subsystem
      settings: PortSchema="{\"entries\":[{\"content\":{\"sides\":[{\"content\":{\"connectorIds\":[]},\"type\":\"ConnectorPlacement.EquallySpacedRectSide\",\"uuid\":\"1dfe2dd4-ea93-4273-8776-58976ddcdaba\"},{\"content\":{\"connectorIds\":[],\"side\":\"RIGHT\"},\"type\":\"ConnectorPlacement.EquallySpacedRectSide\",\"uuid\":\"b7858d1e-d4ca-40f6-96f4-23ffb4bb008a\"},{\"content\":{\"connectorIds\":[\"LConn1\",\"LConn2\",\"LConn3\",\"LConn4\",\"LConn5\",\"LConn6\",\"LConn7\",\"LConn8\",\"LConn9\",\"LConn10\",\"LConn11\",\"LConn12\",\"LConn13\",\"LConn14\"],\"side\":\"TOP\"},\"type\":\"ConnectorPlacement.EquallySpacedRectSide\",\"uuid\":\"2702888d-df0a-4756-9e67-45aa03c3ca26\"},{\"content\":{\"connectorIds\":[\"RConn1\",\"RConn2\",\"RConn3\",\"RConn4\",\"RConn5\",\"RConn6\",\"RConn7\",\"RConn8\",\"RConn9\",\"RConn10\",\"RConn11\",\"RConn12\",\"RConn13\",\"RConn14\"],\"side\":\"BOTTOM\"},\"type\":\"ConnectorPlacement.EquallySpacedRectSide\",\"uuid\":\"cae7576a-06b8-46a3-8430-f7ff5c84a30c\"}]},\"type\":\"ConnectorPlacement.EquallySpacedConnector\",\"uuid\":\"06fdd52a-2b50-4f0d-b8bb-99b205fcd9e0\"}],\"packageUris\":[\"http://schema.mathworks.com/mf0/Connector/R2020b\"],\"version\":\"1.0\"}"
  Pos : PMIOPort  Side=Left
  Neg : PMIOPort  Port=2  Side=Left
  connections:
  Parallel Charge 1/RConn2 -- Busbar  SW 2/LConn1 -- Battery Module 1/RConn2
  Parallel Charge 1/LConn2 -- Busbar  SW 1/RConn1 -- Battery Module 1/LConn1
  Parallel Charge 2/LConn2 -- Busbar  SW 2/RConn1 -- Battery Module 2/LConn1
  Parallel Charge 2/RConn2 -- Busbar  SW 3/LConn1 -- Battery Module 2/RConn2
  Parallel Charge 4/LConn2 -- Battery Module 4/LConn1 -- Busbar  SW 4/RConn1
  Parallel Charge 3/RConn2 -- Battery Module 3/RConn2 -- Busbar  SW 4/LConn1
  Parallel Charge 3/LConn2 -- Busbar  SW 3/RConn1 -- Battery Module 3/LConn1
  Parallel Charge 4/RConn2 -- Busbar  SW 5/LConn1 -- Battery Module 4/RConn2
  Parallel Charge 6/RConn2 -- Busbar  SW 7/LConn1 -- Battery Module 6/RConn2
  Parallel Charge 5/RConn2 -- Busbar  SW 6/LConn1 -- Battery Module 5/RConn2
  Parallel Charge 5/LConn2 -- Busbar  SW 5/RConn1 -- Battery Module 5/LConn1
  Parallel Charge 7/RConn2 -- Busbar  SW 8/LConn1 -- Battery Module 7/RConn2
  Parallel Charge 6/LConn2 -- Busbar  SW 6/RConn1 -- Battery Module 6/LConn1
  Parallel Charge 7/LConn2 -- Busbar  SW 7/RConn1 -- Battery Module 7/LConn1
  Parallel Charge 8/RConn2 -- Busbar  SW 9/LConn1 -- Battery Module 8/RConn2
  Parallel Charge 8/LConn2 -- Busbar  SW 8/RConn1 -- Battery Module 8/LConn1
  Parallel Charge 9/RConn2 -- Battery Module 9/RConn2 -- Busbar  SW 10/LConn1
  Parallel Charge 9/LConn2 -- Busbar  SW 9/RConn1 -- Battery Module 9/LConn1
  Parallel Charge 10/RConn2 -- Busbar  SW 11/LConn1 -- Battery Module 10/RConn2
  Parallel Charge 10/LConn2 -- Busbar  SW 10/RConn1 -- Battery Module 10/LConn1
  Parallel Charge 11/LConn2 -- Busbar  SW 11/RConn1 -- Battery Module 11/LConn1
  Parallel Charge 11/RConn2 -- Busbar  SW 12/LConn1 -- Battery Module 11/RConn2
  Parallel Charge 12/LConn2 -- Busbar  SW 12/RConn1 -- Battery Module 12/LConn1
  Parallel Charge 12/RConn2 -- Busbar  SW 13/LConn1 -- Battery Module 12/RConn2
  Parallel Charge 13/RConn2 -- Busbar  SW 14/LConn1 -- Battery Module 13/RConn2
  Parallel Charge 13/LConn2 -- Busbar  SW 13/RConn1 -- Battery Module 13/LConn1
  Parallel Charge 14/RConn2 -- Busbar  SW 15/LConn1 -- Battery Module 14/RConn2
  Parallel Charge 14/LConn2 -- Busbar  SW 14/RConn1 -- Battery Module 14/LConn1
  Busbar  SW 1/LConn1 -- Pos/RConn1
  Busbar  SW 15/RConn1 -- Neg/RConn1
  Discharge Relay Controller/LConn1 -- Busbar  SW 1/RConn2
  Discharge Relay Controller/LConn2 -- Busbar  SW 2/RConn2
  Busbar  SW 3/RConn2 -- Discharge Relay Controller/LConn3
  Discharge Relay Controller/LConn4 -- Busbar  SW 4/RConn2
  Busbar  SW 5/RConn2 -- Discharge Relay Controller/LConn5
  Busbar  SW 6/RConn2 -- Discharge Relay Controller/LConn6
  Busbar  SW 7/RConn2 -- Discharge Relay Controller/LConn7
  Busbar  SW 8/RConn2 -- Discharge Relay Controller/LConn8
  Discharge Relay Controller/LConn9 -- Busbar  SW 9/RConn2
  Busbar  SW 10/RConn2 -- Discharge Relay Controller/LConn10
  Busbar  SW 11/RConn2 -- Discharge Relay Controller/LConn11
  Discharge Relay Controller/LConn12 -- Busbar  SW 12/RConn2
  Busbar  SW 13/RConn2 -- Discharge Relay Controller/LConn13
  Busbar  SW 14/RConn2 -- Discharge Relay Controller/LConn14
  Busbar  SW 15/RConn2 -- Discharge Relay Controller/LConn15
  Battery Charger 1/LConn1 -- Parallel Charge 1/LConn1
  Battery Charger 1/LConn2 -- Parallel Charge 1/RConn1
  Battery Charger 1/LConn3 -- Parallel Charge 2/LConn1
  Battery Charger 1/LConn4 -- Parallel Charge 2/RConn1
  Battery Charger 1/LConn5 -- Parallel Charge 3/LConn1
  Battery Charger 1/LConn6 -- Parallel Charge 3/RConn1
  Parallel Charge 4/LConn1 -- Battery Charger 2/LConn1
  Battery Charger 2/LConn2 -- Parallel Charge 4/RConn1
  Battery Charger 2/LConn3 -- Parallel Charge 5/LConn1
  Battery Charger 2/LConn4 -- Parallel Charge 5/RConn1
  Battery Charger 2/LConn5 -- Parallel Charge 6/LConn1
  Battery Charger 2/LConn6 -- Parallel Charge 6/RConn1
  Parallel Charge 7/LConn1 -- Battery Charger 3/LConn1
  Battery Charger 3/LConn2 -- Parallel Charge 7/RConn1
  Battery Charger 3/LConn3 -- Parallel Charge 8/LConn1
  Battery Charger 3/LConn4 -- Parallel Charge 8/RConn1
  Battery Charger 3/LConn5 -- Parallel Charge 9/LConn1
  Battery Charger 3/LConn6 -- Parallel Charge 9/RConn1
  Battery Charger 4/LConn1 -- Parallel Charge 10/LConn1
  Battery Charger 4/LConn2 -- Parallel Charge 10/RConn1
  Battery Charger 4/LConn3 -- Parallel Charge 11/LConn1
  Battery Charger 4/LConn4 -- Parallel Charge 11/RConn1
  Battery Charger 4/LConn5 -- Parallel Charge 12/LConn1
  Battery Charger 4/LConn6 -- Parallel Charge 12/RConn1
  Battery Charger 5/LConn1 -- Parallel Charge 13/LConn1
  Battery Charger 5/LConn2 -- Parallel Charge 13/RConn1
  Battery Charger 5/LConn3 -- Parallel Charge 14/LConn1
  Battery Charger 5/LConn4 -- Parallel Charge 14/RConn1
  Parallel Relay Control/RConn1 -- Parallel Charge 1/LConn3
  Parallel Charge 14/LConn3 -- Parallel Relay Control/RConn14
  Parallel Relay Control/RConn2 -- Parallel Charge 2/LConn3
  Parallel Charge 13/LConn3 -- Parallel Relay Control/RConn13
  Parallel Charge 12/LConn3 -- Parallel Relay Control/RConn12
  Parallel Charge 3/LConn3 -- Parallel Relay Control/RConn3
  Parallel Charge 11/LConn3 -- Parallel Relay Control/RConn11
  Parallel Charge 4/LConn3 -- Parallel Relay Control/RConn4
  Parallel Charge 5/LConn3 -- Parallel Relay Control/RConn5
  Parallel Charge 10/LConn3 -- Parallel Relay Control/RConn10
  Parallel Charge 9/LConn3 -- Parallel Relay Control/RConn9
  Parallel Charge 6/LConn3 -- Parallel Relay Control/RConn6
  Parallel Charge 8/LConn3 -- Parallel Relay Control/RConn8
  Parallel Charge 7/LConn3 -- Parallel Relay Control/RConn7
  Battery Module 1/RConn1 -- Thermal Control/LConn1
  Thermal Control/LConn2 -- Battery Module 2/RConn1
  Thermal Control/LConn3 -- Battery Module 3/RConn1
  Battery Module 4/RConn1 -- Thermal Control/LConn4
  Thermal Control/LConn5 -- Battery Module 5/RConn1
  Thermal Control/LConn6 -- Battery Module 6/RConn1
  Thermal Control/LConn7 -- Battery Module 7/RConn1
  Thermal Control/LConn8 -- Battery Module 8/RConn1
  Thermal Control/LConn9 -- Battery Module 9/RConn1
  Thermal Control/LConn10 -- Battery Module 10/RConn1
  Thermal Control/LConn11 -- Battery Module 11/RConn1
  Thermal Control/LConn12 -- Battery Module 12/RConn1
  Thermal Control/LConn13 -- Battery Module 13/RConn1
  Thermal Control/LConn14 -- Battery Module 14/RConn1

== system BatteryFarmTemplate/Battery Conex 1/Battery Charger 1 ==
  DC Voltage Source : fl_lib/Electrical/Electrical Sources/DC Voltage Source  v0=24 V
  DC Voltage Source1 : fl_lib/Electrical/Electrical Sources/DC Voltage Source  v0=24 V
  DC Voltage Source2 : fl_lib/Electrical/Electrical Sources/DC Voltage Source  v0=24 V
  SPST Relay : ee_lib/Switches & Breakers/Relays/SPST Relay  block_choices=ee.enum.controlport.ps  R_closed=0.01 Ohm  G_open=1e-8 1/Ohm  Threshold=0  exposemeasurement=ee.enum.exposemeasurement.hidden  V_rated=5 V  V_energize=75  V_deenergize=25  l_winding=0.08 H  r_winding=12.5 Ohm  g_winding=1e-9 1/Ohm  T_brk_C_S=0 s  T_mak_C_S=0 s  enable_faults=ee.enum.relays.enable.no  fault_action=ee.enum.relays.faultaction.none  fault_types=ee.enum.relays.faultTypes.winding  fault_condition_ps=ee.enum.relays.faultConditionSPSTps.csstuck  r_deg_closed_s=1e-9 Ohm  winding_tau_fault=1e-3 s  tau_fault=1e-3 s  enable_temporal_fault=ee.enum.relays.enable.no  t_fault_stick=1 s  t_fault_ComOpen=1 s  t_fault=1 s  enable_behavioral_fault=ee.enum.relays.enable.no  winding_max_permissible_voltage=inf V  n_fail_on_voltage=1  winding_max_permissible_current=inf A  max_permissible_current=inf A  t_fail_on_current=1 s
      settings: InternalSimscapePortConfiguration="{\"Bottom\":[],\"Left\":[{\"id\":\"PS\",\"label\":\"PS\",\"type\":\"input\"}],\"Right\":[{\"id\":\"S\",\"label\":\"S\",\"type\":\"foundation.electrical.electrical\"},{\"id\":\"COM\",\"label\":\"C\",\"type\":\"foundation.electrical.electrical\"}],\"Top\":[]}"
  SPST Relay1 : ee_lib/Switches & Breakers/Relays/SPST Relay  block_choices=ee.enum.controlport.ps  R_closed=0.01 Ohm  G_open=1e-8 1/Ohm  Threshold=0  exposemeasurement=ee.enum.exposemeasurement.hidden  V_rated=5 V  V_energize=75  V_deenergize=25  l_winding=0.08 H  r_winding=12.5 Ohm  g_winding=1e-9 1/Ohm  T_brk_C_S=0 s  T_mak_C_S=0 s  enable_faults=ee.enum.relays.enable.no  fault_action=ee.enum.relays.faultaction.none  fault_types=ee.enum.relays.faultTypes.winding  fault_condition_ps=ee.enum.relays.faultConditionSPSTps.csstuck  r_deg_closed_s=1e-9 Ohm  winding_tau_fault=1e-3 s  tau_fault=1e-3 s  enable_temporal_fault=ee.enum.relays.enable.no  t_fault_stick=1 s  t_fault_ComOpen=1 s  t_fault=1 s  enable_behavioral_fault=ee.enum.relays.enable.no  winding_max_permissible_voltage=inf V  n_fail_on_voltage=1  winding_max_permissible_current=inf A  max_permissible_current=inf A  t_fail_on_current=1 s
      settings: InternalSimscapePortConfiguration="{\"Bottom\":[],\"Left\":[{\"id\":\"PS\",\"label\":\"PS\",\"type\":\"input\"}],\"Right\":[{\"id\":\"S\",\"label\":\"S\",\"type\":\"foundation.electrical.electrical\"},{\"id\":\"COM\",\"label\":\"C\",\"type\":\"foundation.electrical.electrical\"}],\"Top\":[]}"
  SPST Relay2 : ee_lib/Switches & Breakers/Relays/SPST Relay  block_choices=ee.enum.controlport.ps  R_closed=0.01 Ohm  G_open=1e-8 1/Ohm  Threshold=0  exposemeasurement=ee.enum.exposemeasurement.hidden  V_rated=5 V  V_energize=75  V_deenergize=25  l_winding=0.08 H  r_winding=12.5 Ohm  g_winding=1e-9 1/Ohm  T_brk_C_S=0 s  T_mak_C_S=0 s  enable_faults=ee.enum.relays.enable.no  fault_action=ee.enum.relays.faultaction.none  fault_types=ee.enum.relays.faultTypes.winding  fault_condition_ps=ee.enum.relays.faultConditionSPSTps.csstuck  r_deg_closed_s=1e-9 Ohm  winding_tau_fault=1e-3 s  tau_fault=1e-3 s  enable_temporal_fault=ee.enum.relays.enable.no  t_fault_stick=1 s  t_fault_ComOpen=1 s  t_fault=1 s  enable_behavioral_fault=ee.enum.relays.enable.no  winding_max_permissible_voltage=inf V  n_fail_on_voltage=1  winding_max_permissible_current=inf A  max_permissible_current=inf A  t_fail_on_current=1 s
      settings: InternalSimscapePortConfiguration="{\"Bottom\":[],\"Left\":[{\"id\":\"PS\",\"label\":\"PS\",\"type\":\"input\"}],\"Right\":[{\"id\":\"S\",\"label\":\"S\",\"type\":\"foundation.electrical.electrical\"},{\"id\":\"COM\",\"label\":\"C\",\"type\":\"foundation.electrical.electrical\"}],\"Top\":[]}"
  In 1 : PMIOPort  Side=Left
  Out 1 : PMIOPort  Port=2  Side=Left
  In 2 : PMIOPort  Port=3  Side=Left
  Out 2 : PMIOPort  Port=4  Side=Left
  In 3 : PMIOPort  Port=5  Side=Left
  Out 3 : PMIOPort  Port=6  Side=Left
  Energerize Battery Charger : PMIOPort  Port=7  Side=Right
  connections:
  DC Voltage Source/LConn1 -- SPST Relay/RConn1
  SPST Relay/RConn2 -- In 1/RConn1
  DC Voltage Source/RConn1 -- Out 1/RConn1
  DC Voltage Source1/RConn1 -- Out 2/RConn1
  DC Voltage Source1/LConn1 -- SPST Relay1/RConn1
  SPST Relay1/RConn2 -- In 2/RConn1
  DC Voltage Source2/RConn1 -- Out 3/RConn1
  DC Voltage Source2/LConn1 -- SPST Relay2/RConn1
  SPST Relay2/RConn2 -- In 3/RConn1
  Energerize Battery Charger/RConn1 -- SPST Relay1/LConn1 -- SPST Relay2/LConn1 -- SPST Relay/LConn1

== system BatteryFarmTemplate/Battery Conex 1/Battery Charger 2 ==
  DC Voltage Source : fl_lib/Electrical/Electrical Sources/DC Voltage Source  v0=24 V
  DC Voltage Source1 : fl_lib/Electrical/Electrical Sources/DC Voltage Source  v0=24 V
  DC Voltage Source2 : fl_lib/Electrical/Electrical Sources/DC Voltage Source  v0=24 V
  SPST Relay : ee_lib/Switches & Breakers/Relays/SPST Relay  block_choices=ee.enum.controlport.ps  R_closed=0.01 Ohm  G_open=1e-8 1/Ohm  Threshold=0  exposemeasurement=ee.enum.exposemeasurement.hidden  V_rated=5 V  V_energize=75  V_deenergize=25  l_winding=0.08 H  r_winding=12.5 Ohm  g_winding=1e-9 1/Ohm  T_brk_C_S=0 s  T_mak_C_S=0 s  enable_faults=ee.enum.relays.enable.no  fault_action=ee.enum.relays.faultaction.none  fault_types=ee.enum.relays.faultTypes.winding  fault_condition_ps=ee.enum.relays.faultConditionSPSTps.csstuck  r_deg_closed_s=1e-9 Ohm  winding_tau_fault=1e-3 s  tau_fault=1e-3 s  enable_temporal_fault=ee.enum.relays.enable.no  t_fault_stick=1 s  t_fault_ComOpen=1 s  t_fault=1 s  enable_behavioral_fault=ee.enum.relays.enable.no  winding_max_permissible_voltage=inf V  n_fail_on_voltage=1  winding_max_permissible_current=inf A  max_permissible_current=inf A  t_fail_on_current=1 s
      settings: InternalSimscapePortConfiguration="{\"Bottom\":[],\"Left\":[{\"id\":\"PS\",\"label\":\"PS\",\"type\":\"input\"}],\"Right\":[{\"id\":\"S\",\"label\":\"S\",\"type\":\"foundation.electrical.electrical\"},{\"id\":\"COM\",\"label\":\"C\",\"type\":\"foundation.electrical.electrical\"}],\"Top\":[]}"
  SPST Relay1 : ee_lib/Switches & Breakers/Relays/SPST Relay  block_choices=ee.enum.controlport.ps  R_closed=0.01 Ohm  G_open=1e-8 1/Ohm  Threshold=0  exposemeasurement=ee.enum.exposemeasurement.hidden  V_rated=5 V  V_energize=75  V_deenergize=25  l_winding=0.08 H  r_winding=12.5 Ohm  g_winding=1e-9 1/Ohm  T_brk_C_S=0 s  T_mak_C_S=0 s  enable_faults=ee.enum.relays.enable.no  fault_action=ee.enum.relays.faultaction.none  fault_types=ee.enum.relays.faultTypes.winding  fault_condition_ps=ee.enum.relays.faultConditionSPSTps.csstuck  r_deg_closed_s=1e-9 Ohm  winding_tau_fault=1e-3 s  tau_fault=1e-3 s  enable_temporal_fault=ee.enum.relays.enable.no  t_fault_stick=1 s  t_fault_ComOpen=1 s  t_fault=1 s  enable_behavioral_fault=ee.enum.relays.enable.no  winding_max_permissible_voltage=inf V  n_fail_on_voltage=1  winding_max_permissible_current=inf A  max_permissible_current=inf A  t_fail_on_current=1 s
      settings: InternalSimscapePortConfiguration="{\"Bottom\":[],\"Left\":[{\"id\":\"PS\",\"label\":\"PS\",\"type\":\"input\"}],\"Right\":[{\"id\":\"S\",\"label\":\"S\",\"type\":\"foundation.electrical.electrical\"},{\"id\":\"COM\",\"label\":\"C\",\"type\":\"foundation.electrical.electrical\"}],\"Top\":[]}"
  SPST Relay2 : ee_lib/Switches & Breakers/Relays/SPST Relay  block_choices=ee.enum.controlport.ps  R_closed=0.01 Ohm  G_open=1e-8 1/Ohm  Threshold=0  exposemeasurement=ee.enum.exposemeasurement.hidden  V_rated=5 V  V_energize=75  V_deenergize=25  l_winding=0.08 H  r_winding=12.5 Ohm  g_winding=1e-9 1/Ohm  T_brk_C_S=0 s  T_mak_C_S=0 s  enable_faults=ee.enum.relays.enable.no  fault_action=ee.enum.relays.faultaction.none  fault_types=ee.enum.relays.faultTypes.winding  fault_condition_ps=ee.enum.relays.faultConditionSPSTps.csstuck  r_deg_closed_s=1e-9 Ohm  winding_tau_fault=1e-3 s  tau_fault=1e-3 s  enable_temporal_fault=ee.enum.relays.enable.no  t_fault_stick=1 s  t_fault_ComOpen=1 s  t_fault=1 s  enable_behavioral_fault=ee.enum.relays.enable.no  winding_max_permissible_voltage=inf V  n_fail_on_voltage=1  winding_max_permissible_current=inf A  max_permissible_current=inf A  t_fail_on_current=1 s
      settings: InternalSimscapePortConfiguration="{\"Bottom\":[],\"Left\":[{\"id\":\"PS\",\"label\":\"PS\",\"type\":\"input\"}],\"Right\":[{\"id\":\"S\",\"label\":\"S\",\"type\":\"foundation.electrical.electrical\"},{\"id\":\"COM\",\"label\":\"C\",\"type\":\"foundation.electrical.electrical\"}],\"Top\":[]}"
  In 1 : PMIOPort  Side=Left
  Out 1 : PMIOPort  Port=2  Side=Left
  In 2 : PMIOPort  Port=3  Side=Left
  Out 2 : PMIOPort  Port=4  Side=Left
  In 3 : PMIOPort  Port=5  Side=Left
  Out 3 : PMIOPort  Port=6  Side=Left
  Energerize Battery Charger : PMIOPort  Port=7  Side=Right
  connections:
  DC Voltage Source/LConn1 -- SPST Relay/RConn1
  SPST Relay/RConn2 -- In 1/RConn1
  DC Voltage Source/RConn1 -- Out 1/RConn1
  DC Voltage Source1/RConn1 -- Out 2/RConn1
  DC Voltage Source1/LConn1 -- SPST Relay1/RConn1
  SPST Relay1/RConn2 -- In 2/RConn1
  DC Voltage Source2/RConn1 -- Out 3/RConn1
  DC Voltage Source2/LConn1 -- SPST Relay2/RConn1
  SPST Relay2/RConn2 -- In 3/RConn1
  SPST Relay1/LConn1 -- Energerize Battery Charger/RConn1 -- SPST Relay/LConn1 -- SPST Relay2/LConn1
